simulink model "Simulation_6DOFTesting03"  (R2024a)
settings: Solver=ode4  StartTime=initial_time  StopTime=final_time  FixedStep=timestep  RelTol=1e-3
values from neighbouring files (symbols this model uses):
  aEarth = 0    [CodeTesting_6DOF.m]    (also in Constants_6DOF.m = 6378137; Constants_6DOFTesting.m = 6378137)
  alphaArray = [-30, -25, -20, -15, -10, -5, 0, 5, 10, 15, 20, 25, 30]    [CodeTesting_6DOF.m]    (also in Constants_6DOF.m; Constants_6DOFTesting.m)
  altitudeArray = [0, 1000, 2000, 3000, 4000, 5000, 6000, 7000, 8000, 9000, 10000, 15000, 20000,      25000, 30000, 35000, 40000, 45000, 50000, 55000, 60000]    [CodeTesting_6DOF.m]    (also in Constants_6DOF.m; Constants_6DOFTesting.m)
  bEarth = 0    [CodeTesting_6DOF.m]    (also in Constants_6DOF.m = 6356752.3; Constants_6DOFTesting.m = 6356752.3)
  cD_3DArray = zeros(numAoAs, numMachs, numAltitudes)    [CodeTesting_6DOF.m]    (also in Constants_6DOF.m; Constants_6DOFTesting.m)
  cL_3DArray = zeros(numAoAs, numMachs, numAltitudes)    [CodeTesting_6DOF.m]    (also in Constants_6DOF.m; Constants_6DOFTesting.m)
  densityList = rhoList    [CodeTesting_6DOF.m]    (also in Constants_6DOF.m = usAtmosphere.x_; Constants_6DOFTesting.m = usAtmosphere.x_)
  height0 = 0    [Constants_6DOF.m]    (also in Constants_6DOFTesting.m = 5000)
  heightsList = usAtmosphere.Z    [CodeTesting_6DOF.m]    (also in Constants_6DOF.m; Constants_6DOFTesting.m)
  inertialPitch0 = deg2rad(inertialPitch0)    [Constants_6DOFTesting.m]
  inertialRoll0 = deg2rad(inertialRoll0)    [Constants_6DOFTesting.m]
  inertialYaw0 = deg2rad(inertialYaw0)    [Constants_6DOFTesting.m]
  initQuatVector0 = [e0; e1; e2; e3]    [Constants_6DOFTesting.m]
  Ixx = 10    [CodeTesting_6DOF.m]    (also in Constants_6DOF.m; Constants_6DOFTesting.m = 4.88094462)
  Ixz = 10    [CodeTesting_6DOF.m]    (also in Constants_6DOF.m = 1; Constants_6DOFTesting.m = 4.88094462)
  Iyy = 10    [CodeTesting_6DOF.m]    (also in Constants_6DOF.m; Constants_6DOFTesting.m = 4.88094462)
  Izz = 10    [CodeTesting_6DOF.m]    (also in Constants_6DOF.m; Constants_6DOFTesting.m = 4.88094462)
  latitude0 = pi/4    (= 0.785398163397)    [CodeTesting_6DOF.m]    (also in Constants_6DOF.m = deg2rad(latitude0); Constants_6DOFTesting.m = deg2rad(latitude0))
  longitude0 = pi/4    (= 0.785398163397)    [CodeTesting_6DOF.m]    (also in Constants_6DOF.m = deg2rad(longitude0); Constants_6DOFTesting.m = deg2rad(longitude0))
  m0 = 10    [CodeTesting_6DOF.m]    (also in Constants_6DOF.m = 50; Constants_6DOFTesting.m = 14.5939029)
  machArray = [0.5, 1.0, 1.5, 2.0, 2.5, 3.0, 3.5, 4.0, 4.5, 5.0, 5.5, 6.0, 6.5, 7.0, 7.5, 8.0,      8.5, 9.0, 9.5, 10.0]    [CodeTesting_6DOF.m]    (also in Constants_6DOF.m; Constants_6DOFTesting.m)
  omegaEarth = omega_earth    (= 7.2921159e-05)    [CodeTesting_6DOF.m]    (also in Constants_6DOF.m; Constants_6DOFTesting.m)
  p0Body = deg2rad(p0Body)    [Constants_6DOFTesting.m]
  pitchCharacteristicLength = 0.0    (= 0)    [Constants_6DOFTesting.m]
  q0Body = deg2rad(q0Body)    [Constants_6DOFTesting.m]
  r0Body = deg2rad(r0Body)    [Constants_6DOFTesting.m]
  rEarth = r_earth    (= 6371008.8)    [CodeTesting_6DOF.m]    (also in Constants_6DOF.m; Constants_6DOFTesting.m)
  rollCharacteristicLength = 0.0    (= 0)    [Constants_6DOFTesting.m]
  temperatureList = usAtmosphere.T    [CodeTesting_6DOF.m]    (also in Constants_6DOF.m; Constants_6DOFTesting.m)
  u0Body = 304.8    [Constants_6DOFTesting.m]
  v0Body = 0    [Constants_6DOFTesting.m]
  w0Body = -1 * w0Body    (= 0)    [Constants_6DOFTesting.m]
  wingArea = 0    [CodeTesting_6DOF.m]    (also in Constants_6DOF.m = 50; Constants_6DOFTesting.m = 0.09290304)
  yawCharacteristicLength = 0.0    (= 0)    [Constants_6DOFTesting.m]
undefined symbols (not defined in the file or in its folder): inertialX0, inertialY0, inertialZ0
libraries: simulink_extras x24
(part 1 of 2)
settings Model: Creator=641893  LastModifiedBy=641893

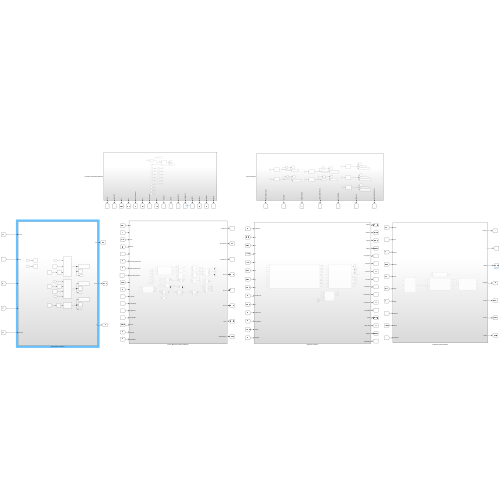
[thumbnail: Simulink's stored preview of the top-level diagram]
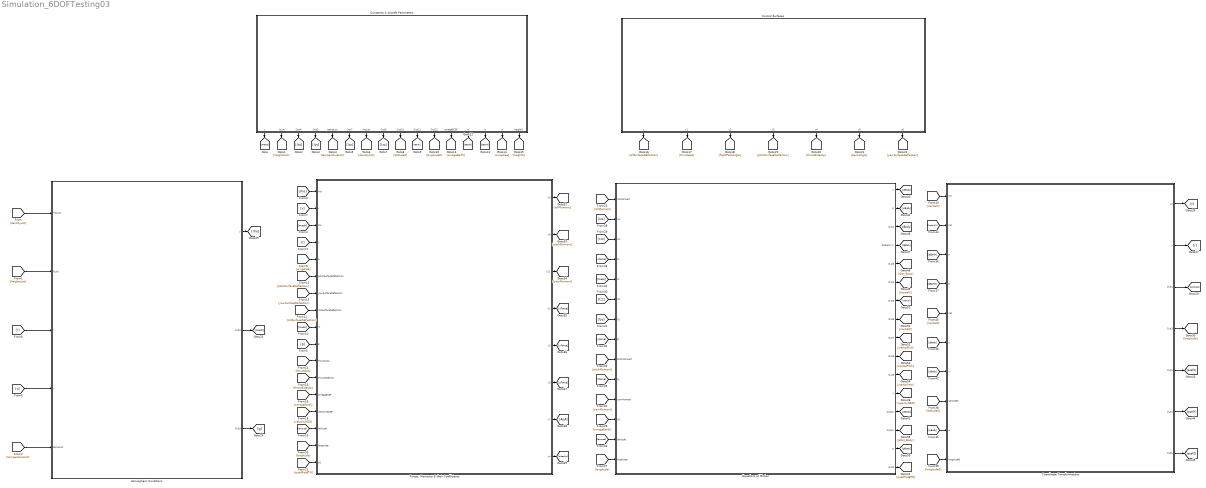
== system Simulation_6DOFTesting03 ==
  Atmospheric Conditions : Subsystem
  Constants & Aircraft Parameters : Subsystem
  Control Surfaces : Subsystem
  Coordinate Transformations : Subsystem
  Equations of Motion : Subsystem
  "Forces, Moments & their Coefficients" : Subsystem
  wires:
  Constants & Aircraft Parameters/1(y) -> [mass]
  Constants & Aircraft Parameters/2(hList) -> [heightsList]
  Constants & Aircraft Parameters/3(Out4) -> [Ixx]
  Constants & Aircraft Parameters/4(Out5) -> [Iyy]
  Constants & Aircraft Parameters/5(tempList) -> [temperatureList]
  Constants & Aircraft Parameters/6(Out7) -> [Izz]
  Constants & Aircraft Parameters/7(rhoList) -> [densityList]
  Constants & Aircraft Parameters/8(Out9) -> [Ixz]
  Constants & Aircraft Parameters/9(Out10) -> [latitude0]
  Constants & Aircraft Parameters/10(Out11) -> [rEarth]
  Constants & Aircraft Parameters/11(Out12) -> [longitude0]
  Constants & Aircraft Parameters/12(omegaECEF) -> [omegaEarth]
  Constants & Aircraft Parameters/13(a) -> [aEarth]
  Constants & Aircraft Parameters/14(b) -> [bEarth]
  Constants & Aircraft Parameters/15(A) -> [wingArea]
  Constants & Aircraft Parameters/16(height0) -> [height0]
  Control Surfaces/1(y) -> [rollSurfaceDeflection]
  Control Surfaces/2(y1) -> [thrustAoA]
  Control Surfaces/4(y3) -> [pitchSurfaceDeflection]
  Control Surfaces/3(y2) -> [flightPathAngle]
  Control Surfaces/5(y4) -> [thrustSideslip]
  Control Surfaces/6(y5) -> [bankAngle]
  Control Surfaces/7(y6) -> [yawSurfaceDeflection]
  [densityList] -> Atmospheric Conditions/1(rhoList)
  [heightsList] -> Atmospheric Conditions/2(hList)
  [temperatureList] -> Atmospheric Conditions/5(tempList)
  Atmospheric Conditions/1(y) -> [rho]
  Atmospheric Conditions/2(Out2) -> [mach]
  Atmospheric Conditions/3(Out3) -> [g]
  [rho] -> "Forces, Moments & their Coefficients"/1(rho)
  [mach] -> "Forces, Moments & their Coefficients"/3(In4)
  [g] -> "Forces, Moments & their Coefficients"/10(g)
  Coordinate Transformations/1(y4) -> [v]
  [v] -> Atmospheric Conditions/4(v)
  [v] -> "Forces, Moments & their Coefficients"/2(v)
  Coordinate Transformations/2(y) -> [r]
  [r] -> Atmospheric Conditions/3(r)
  [wingArea] -> "Forces, Moments & their Coefficients"/5(A)
  [mass] -> "Forces, Moments & their Coefficients"/9(m)
  [rollSurfaceDeflection] -> "Forces, Moments & their Coefficients"/8(rollSurfaceDeflection)
  [pitchSurfaceDeflection] -> "Forces, Moments & their Coefficients"/6(pitchSurfaceDeflection)
  [yawSurfaceDeflection] -> "Forces, Moments & their Coefficients"/7(yawSurfaceDeflection)
  [thrustAoA] -> "Forces, Moments & their Coefficients"/11(thrustAoA)
  [thrustSideslip] -> "Forces, Moments & their Coefficients"/12(thrustSideslip)
  [omegaEarth] -> "Forces, Moments & their Coefficients"/13(omegaECEF)
  [r] -> "Forces, Moments & their Coefficients"/4(y)
  Equations of Motion/12(y) -> [velocityNED]
  [velocityNED] -> "Forces, Moments & their Coefficients"/14(velocityECEF)
  Coordinate Transformations/3(Out1) -> [latitude]
  Coordinate Transformations/4(Out3) -> [longitude]
  [latitude] -> "Forces, Moments & their Coefficients"/15(latitude)
  [longitude] -> "Forces, Moments & their Coefficients"/16(longitude)
  Equations of Motion/16(Out2) -> [quadRotBTN]
  [quadRotBTN] -> "Forces, Moments & their Coefficients"/17(In1)
  "Forces, Moments & their Coefficients"/1(y5) -> [rollMoment]
  "Forces, Moments & their Coefficients"/2(y8) -> [pitchMoment]
  "Forces, Moments & their Coefficients"/3(y11) -> [yawMoment]
  [rollMoment] -> Equations of Motion/1(rollMoment)
  [pitchMoment] -> Equations of Motion/9(pitchMoment)
  [yawMoment] -> Equations of Motion/11(yawMoment)
  [omegaEarth] -> Equations of Motion/12(In1)
  [latitude] -> Equations of Motion/13(latitude)
  [longitude] -> Equations of Motion/14(longitude)
  [Ixx] -> Equations of Motion/2(Ixx)
  [Ixz] -> Equations of Motion/3(Ixz)
  [Izz] -> Equations of Motion/6(Izz)
  [Iyy] -> Equations of Motion/7(Iyy)
  [mass] -> Equations of Motion/5(m)
  "Forces, Moments & their Coefficients"/4(y1) -> [xForce]
  "Forces, Moments & their Coefficients"/5(y2) -> [yForce]
  "Forces, Moments & their Coefficients"/6(y3) -> [zForce]
  [xForce] -> Equations of Motion/4(Fx)
  [yForce] -> Equations of Motion/8(Fy)
  [zForce] -> Equations of Motion/10(Fz)
  "Forces, Moments & their Coefficients"/7(y7) -> [AoA]
  "Forces, Moments & their Coefficients"/8(y4) -> [sideslip]
  [aEarth] -> Coordinate Transformations/3(a)
  [bEarth] -> Coordinate Transformations/4(b)
  [latitude0] -> Coordinate Transformations/8(latitude0)
  [longitude0] -> Coordinate Transformations/10(longitude0)
  Equations of Motion/1(u) -> [uBody]
  Equations of Motion/2(w) -> [wBody]
  [uBody] -> Coordinate Transformations/6(u)
  [wBody] -> Coordinate Transformations/9(w)
  Equations of Motion/13(Out10) -> [vBody]
  [vBody] -> Coordinate Transformations/7(v)
  Equations of Motion/3(Out1) -> [rBody]
  Equations of Motion/4(Radians in) -> [qBody]
  Equations of Motion/5(Out3) -> [rDot_Body]
  Equations of Motion/6(Out4) -> [inertialX]
  Equations of Motion/7(Out5) -> [inertialY]
  Equations of Motion/8(Out6) -> [inertialZ]
  Equations of Motion/9(Out7) -> [inertialRoll]
  Equations of Motion/10(Out8) -> [inertialPitch]
  Equations of Motion/11(Out9) -> [inertialYaw]
  Equations of Motion/14(Out11) -> [pDot_Body]
  Equations of Motion/15(p) -> [pBody]
  [inertialX] -> Coordinate Transformations/1(In1)
  [inertialY] -> Coordinate Transformations/2(In3)
  [inertialZ] -> Coordinate Transformations/5(In8)
  Coordinate Transformations/5(Out2) -> [ecefX]
  Coordinate Transformations/6(Out4) -> [ecefY]
  Coordinate Transformations/7(Out5) -> [ecefZ]

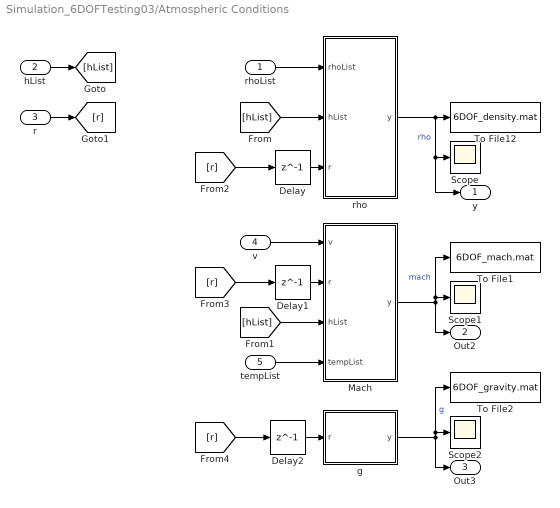
== system Simulation_6DOFTesting03/Atmospheric Conditions ==
  rhoList : Inport
  hList : Inport  Port=2
  r : Inport  Port=3
  v : Inport  Port=4
  tempList : Inport  Port=5
  Delay : Delay  DelayLength=1  InitialCondition=0
  Delay1 : Delay  DelayLength=1  InitialCondition=0
  Delay2 : Delay  DelayLength=1  InitialCondition=0
  Mach : MATLAB Function  TreatAsAtomicUnit=on
  Scope : Scope
  Scope1 : Scope
  Scope2 : Scope
  To File1 : ToFile  Filename=6DOF_mach.mat
  To File12 : ToFile  Filename=6DOF_density.mat
  To File2 : ToFile  Filename=6DOF_gravity.mat
  g : MATLAB Function  TreatAsAtomicUnit=on
  rho : MATLAB Function  TreatAsAtomicUnit=on
  y : Outport
  Out2 : Outport  Port=2
  Out3 : Outport  Port=3
  wires:
  rho/1(y) -> Scope/1, y/1, To File12/1  "rho"
  Mach/1(y) -> To File1/1, Scope1/1, Out2/1  "mach"
  g/1(y) -> Out3/1, To File2/1, Scope2/1  "g"
  v/1 -> Mach/1(v)
  tempList/1 -> Mach/4(tempList)
  r/1 -> [r]
  rhoList/1 -> rho/1(rhoList)
  hList/1 -> [hList]
  [hList] -> rho/2(hList)
  [hList] -> Mach/3(hList)
  Delay/1 -> rho/3(r)
  Delay1/1 -> Mach/2(r)
  Delay2/1 -> g/1(r)
  [r] -> Delay/1
  [r] -> Delay1/1
  [r] -> Delay2/1

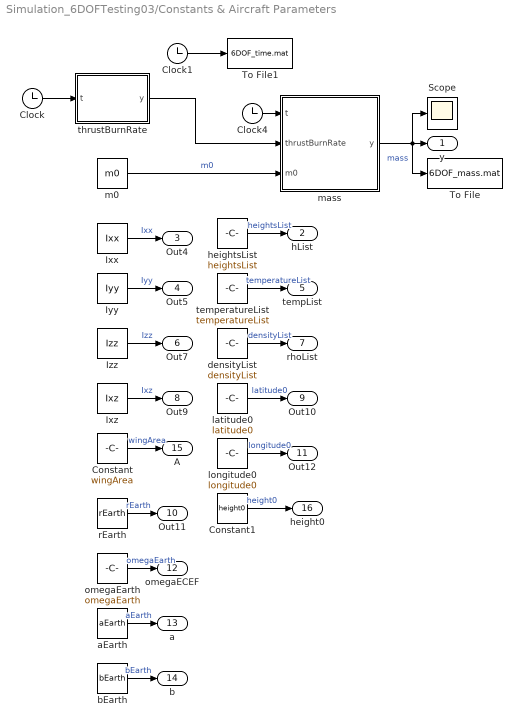
== system Simulation_6DOFTesting03/Constants & Aircraft Parameters ==
  Clock : Clock
  Clock1 : Clock
  Clock4 : Clock
  Constant : Constant  Value=wingArea
  Constant1 : Constant  Value=height0
  Ixx : Constant  Value=Ixx
  Ixz : Constant  Value=Ixz
  Iyy : Constant  Value=Iyy
  Izz : Constant  Value=Izz
  Scope : Scope
  To File : ToFile  Filename=6DOF_mass.mat
  To File1 : ToFile  Filename=6DOF_time.mat
  aEarth : Constant  Value=aEarth
  bEarth : Constant  Value=bEarth
  densityList : Constant  Value=densityList
  heightsList : Constant  Value=heightsList
  latitude0 : Constant  Value=latitude0
  longitude0 : Constant  Value=longitude0
  m0 : Constant  Value=m0
  mass : MATLAB Function  TreatAsAtomicUnit=on
  omegaEarth : Constant  Value=omegaEarth
  rEarth : Constant  Value=rEarth
  temperatureList : Constant  Value=temperatureList
  thrustBurnRate : MATLAB Function  TreatAsAtomicUnit=on
  y : Outport
  hList : Outport  Port=2
  Out4 : Outport  Port=3
  Out5 : Outport  Port=4
  tempList : Outport  Port=5
  Out7 : Outport  Port=6
  rhoList : Outport  Port=7
  Out9 : Outport  Port=8
  Out10 : Outport  Port=9
  Out11 : Outport  Port=10
  Out12 : Outport  Port=11
  omegaECEF : Outport  Port=12
  a : Outport  Port=13
  b : Outport  Port=14
  A : Outport  Port=15
  height0 : Outport  Port=16
  wires:
  m0/1 -> mass/3(m0)  "m0"
  Clock4/1 -> mass/1(t)
  heightsList/1 -> hList/1  "heightsList"
  Clock/1 -> thrustBurnRate/1(t)
  omegaEarth/1 -> omegaECEF/1  "omegaEarth"
  thrustBurnRate/1(y) -> mass/2(thrustBurnRate)
  rEarth/1 -> Out11/1  "rEarth"
  latitude0/1 -> Out10/1  "latitude0"
  mass/1(y) -> To File/1, Scope/1, y/1  "mass"
  aEarth/1 -> a/1  "aEarth"
  densityList/1 -> rhoList/1  "densityList"
  longitude0/1 -> Out12/1  "longitude0"
  bEarth/1 -> b/1  "bEarth"
  Izz/1 -> Out7/1  "Izz"
  Ixz/1 -> Out9/1  "Ixz"
  Ixx/1 -> Out4/1  "Ixx"
  temperatureList/1 -> tempList/1  "temperatureList"
  Iyy/1 -> Out5/1  "Iyy"
  Constant/1 -> A/1  "wingArea"
  Clock1/1 -> To File1/1
  Constant1/1 -> height0/1  "height0"

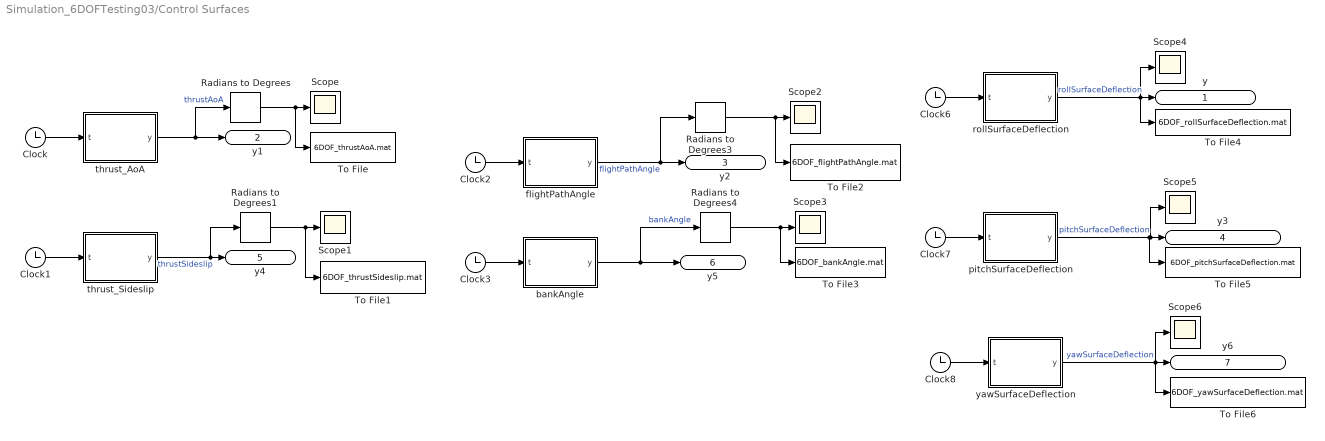
== system Simulation_6DOFTesting03/Control Surfaces ==
  Clock{,1..3,6..8} (7 alike) : Clock
  Radians to Degrees{,1,3..4} (4 alike) : simulink_extras/Transformations/Radians to Degrees
  Scope{,1..6} (7 alike) : Scope
  To File : ToFile  Filename=6DOF_thrustAoA.mat
  To File1 : ToFile  Filename=6DOF_thrustSideslip.mat
  To File2 : ToFile  Filename=6DOF_flightPathAngle.mat
  To File3 : ToFile  Filename=6DOF_bankAngle.mat
  To File4 : ToFile  Filename=6DOF_rollSurfaceDeflection.mat
  To File5 : ToFile  Filename=6DOF_pitchSurfaceDeflection.mat
  To File6 : ToFile  Filename=6DOF_yawSurfaceDeflection.mat
  bankAngle : MATLAB Function  TreatAsAtomicUnit=on
  flightPathAngle : MATLAB Function  TreatAsAtomicUnit=on
  pitchSurfaceDeflection : MATLAB Function  TreatAsAtomicUnit=on
  rollSurfaceDeflection : MATLAB Function  TreatAsAtomicUnit=on
  thrust_AoA : MATLAB Function  TreatAsAtomicUnit=on
  thrust_Sideslip : MATLAB Function  TreatAsAtomicUnit=on
  yawSurfaceDeflection : MATLAB Function  TreatAsAtomicUnit=on
  y : Outport
  y1 : Outport  Port=2
  y2 : Outport  Port=3
  y3 : Outport  Port=4
  y4 : Outport  Port=5
  y5 : Outport  Port=6
  y6 : Outport  Port=7
  wires:
  Clock8/1 -> yawSurfaceDeflection/1(t)
  rollSurfaceDeflection/1(y) -> Scope4/1, y/1, To File4/1  "rollSurfaceDeflection"
  Clock1/1 -> thrust_Sideslip/1(t)
  bankAngle/1(y) -> Radians to Degrees4/1, y5/1  "bankAngle"
  Clock6/1 -> rollSurfaceDeflection/1(t)
  Clock7/1 -> pitchSurfaceDeflection/1(t)
  pitchSurfaceDeflection/1(y) -> To File5/1, Scope5/1, y3/1  "pitchSurfaceDeflection"
  Clock2/1 -> flightPathAngle/1(t)
  thrust_AoA/1(y) -> Radians to Degrees/1, y1/1  "thrustAoA"
  Clock/1 -> thrust_AoA/1(t)
  Clock3/1 -> bankAngle/1(t)
  thrust_Sideslip/1(y) -> Radians to Degrees1/1, y4/1  "thrustSideslip"
  flightPathAngle/1(y) -> Radians to Degrees3/1, y2/1  "flightPathAngle"
  yawSurfaceDeflection/1(y) -> Scope6/1, y6/1, To File6/1  "yawSurfaceDeflection"
  Radians to Degrees/1 -> To File/1, Scope/1
  Radians to Degrees1/1 -> To File1/1, Scope1/1
  Radians to Degrees3/1 -> To File2/1, Scope2/1
  Radians to Degrees4/1 -> Scope3/1, To File3/1

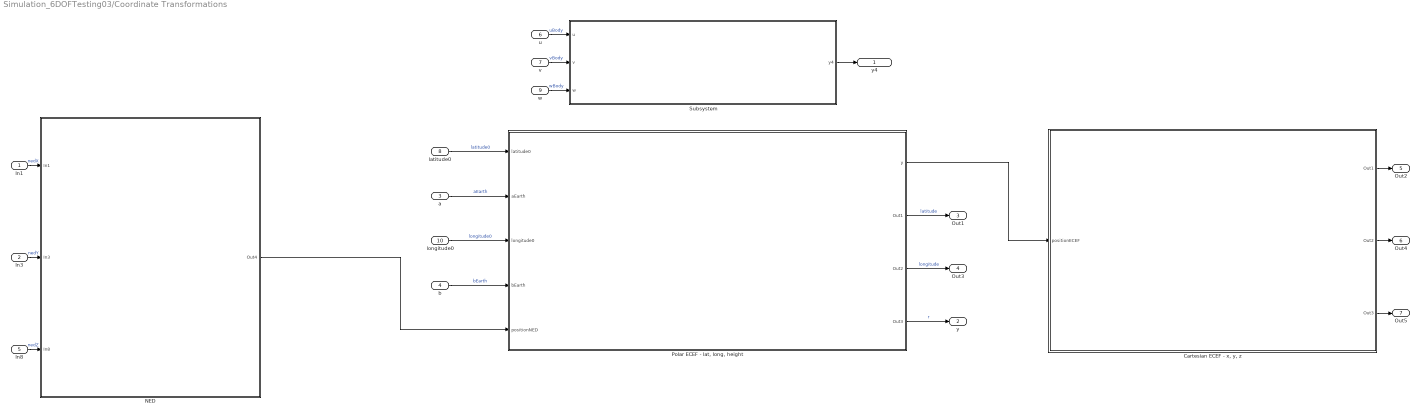
== system Simulation_6DOFTesting03/Coordinate Transformations ==
  In1 : Inport
  In3 : Inport  Port=2
  a : Inport  Port=3
  b : Inport  Port=4
  In8 : Inport  Port=5
  u : Inport  Port=6
  v : Inport  Port=7
  latitude0 : Inport  Port=8
  w : Inport  Port=9
  longitude0 : Inport  Port=10
  "Cartesian ECEF - x, y, z" : Subsystem
  NED : Subsystem
  "Polar ECEF - lat, long, height" : Subsystem
  Subsystem : Subsystem
  y4 : Outport
  y : Outport  Port=2
  Out1 : Outport  Port=3
  Out3 : Outport  Port=4
  Out2 : Outport  Port=5
  Out4 : Outport  Port=6
  Out5 : Outport  Port=7
  wires:
  b/1 -> "Polar ECEF - lat, long, height"/4(bEarth)  "bEarth"
  longitude0/1 -> "Polar ECEF - lat, long, height"/3(longitude0)  "longitude0"
  latitude0/1 -> "Polar ECEF - lat, long, height"/1(latitude0)  "latitude0"
  a/1 -> "Polar ECEF - lat, long, height"/2(aEarth)  "aEarth"
  NED/1(Out4) -> "Polar ECEF - lat, long, height"/5(positionNED)
  In1/1 -> NED/1(In1)  "nedX"
  In3/1 -> NED/2(In3)  "nedY"
  In8/1 -> NED/3(In8)  "nedZ"
  "Polar ECEF - lat, long, height"/1(y) -> "Cartesian ECEF - x, y, z"/1(positionECEF)
  u/1 -> Subsystem/1(u)  "uBody"
  v/1 -> Subsystem/2(v)  "vBody"
  w/1 -> Subsystem/3(w)  "wBody"
  Subsystem/1(y4) -> y4/1
  "Polar ECEF - lat, long, height"/3(Out2) -> Out3/1  "longitude"
  "Polar ECEF - lat, long, height"/2(Out1) -> Out1/1  "latitude"
  "Cartesian ECEF - x, y, z"/3(Out3) -> Out5/1
  "Cartesian ECEF - x, y, z"/2(Out2) -> Out4/1
  "Cartesian ECEF - x, y, z"/1(Out1) -> Out2/1
  "Polar ECEF - lat, long, height"/4(Out3) -> y/1  "r"

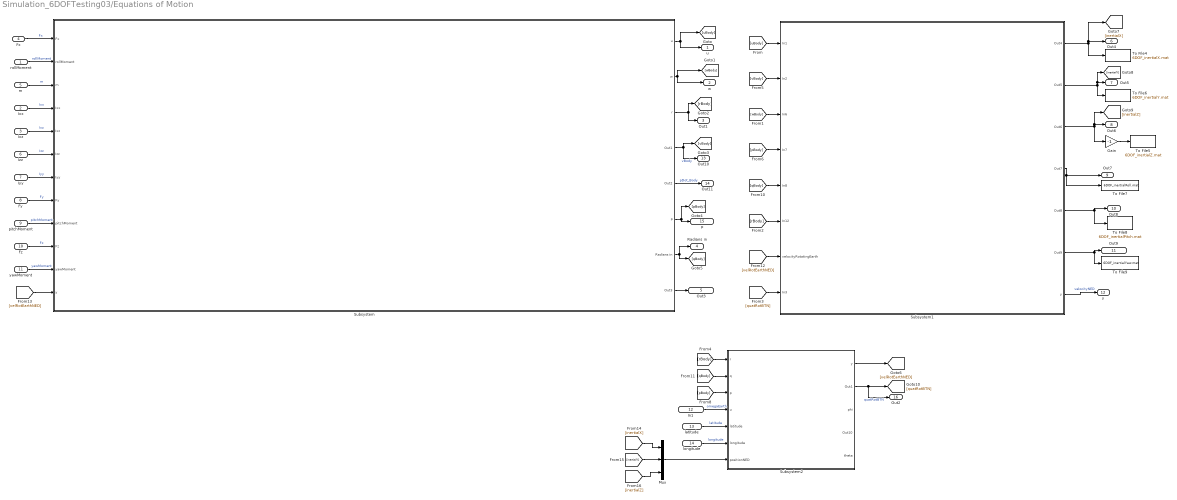
== system Simulation_6DOFTesting03/Equations of Motion ==
  rollMoment : Inport
  Ixx : Inport  Port=2
  Ixz : Inport  Port=3
  Fx : Inport  Port=4
  m : Inport  Port=5
  Izz : Inport  Port=6
  Iyy : Inport  Port=7
  Fy : Inport  Port=8
  pitchMoment : Inport  Port=9
  Fz : Inport  Port=10
  yawMoment : Inport  Port=11
  In1 : Inport  Port=12
  latitude : Inport  Port=13
  longitude : Inport  Port=14
  Gain : Gain  Gain=-1
  Mux : Mux  Inputs=3
  Subsystem : Subsystem
  Subsystem1 : Subsystem
  Subsystem2 : Subsystem
  To File4 : ToFile  Filename=6DOF_inertialX.mat
  To File5 : ToFile  Filename=6DOF_inertialZ.mat
  To File6 : ToFile  Filename=6DOF_inertialY.mat
  To File7 : ToFile  Filename=6DOF_inertialRoll.mat
  To File8 : ToFile  Filename=6DOF_inertialPitch.mat
  To File9 : ToFile  Filename=6DOF_inertialYaw.mat
  u : Outport
  w : Outport  Port=2
  Out1 : Outport  Port=3
  Radians in : Outport  Port=4
  Out3 : Outport  Port=5
  Out4 : Outport  Port=6
  Out5 : Outport  Port=7
  Out6 : Outport  Port=8
  Out7 : Outport  Port=9
  Out8 : Outport  Port=10
  Out9 : Outport  Port=11
  y : Outport  Port=12
  Out10 : Outport  Port=13
  Out11 : Outport  Port=14
  p : Outport  Port=15
  Out2 : Outport  Port=16
  wires:
  Fx/1 -> Subsystem/1(Fx)  "Fx"
  rollMoment/1 -> Subsystem/2(rollMoment)  "rollMoment"
  m/1 -> Subsystem/3(m)  "m"
  Ixx/1 -> Subsystem/4(Ixx)  "Ixx"
  Ixz/1 -> Subsystem/5(Ixz)  "Ixz"
  Izz/1 -> Subsystem/6(Izz)  "Izz"
  Iyy/1 -> Subsystem/7(Iyy)  "Iyy"
  Fy/1 -> Subsystem/8(Fy)  "Fy"
  pitchMoment/1 -> Subsystem/9(pitchMoment)  "pitchMoment"
  Fz/1 -> Subsystem/10(Fz)  "Fz"
  yawMoment/1 -> Subsystem/11(yawMoment)  "yawMoment"
  Subsystem/1(u) -> [uBody], u/1
  Subsystem/2(w) -> [wBody], w/1
  Subsystem/3(r) -> [rBody], Out1/1
  Subsystem/8(Out3) -> Out3/1
  Subsystem1/1(Out4) -> Out4/1, [inertialX], To File4/1
  Subsystem1/2(Out5) -> Out5/1, [inertialY], To File6/1
  Subsystem1/3(Out6) -> Out6/1, [inertialZ], Gain/1
  Subsystem1/4(Out7) -> To File7/1, Out7/1
  Subsystem1/6(Out9) -> Out9/1, To File9/1
  In1/1 -> Subsystem2/4(u)  "omegaEarth"
  Subsystem2/1(y) -> [velRotEarthNED]
  latitude/1 -> Subsystem2/5(latitude)  "latitude"
  longitude/1 -> Subsystem2/6(longitude)  "longitude"
  Mux/1 -> Subsystem2/7(positionNED)
  Gain/1 -> To File5/1
  Subsystem1/7(y) -> y/1  "velocityNED"
  [uBody] -> Subsystem1/1(In1)
  [wBody] -> Subsystem1/3(In6)
  [rBody] -> Subsystem1/6(In12)
  [rBody] -> Subsystem2/1(r)
  Subsystem/4(Out1) -> [vBody], Out10/1  "vBody"
  [vBody] -> Subsystem1/2(In2)
  Subsystem/6(p) -> p/1, [pBody]
  [pBody] -> Subsystem1/4(In7)
  [pBody] -> Subsystem2/3(p)
  Subsystem/5(Out2) -> Out11/1  "pDot_Body"
  Subsystem/7(Radians in) -> [qBody], Radians in/1
  [qBody] -> Subsystem1/5(In8)
  [qBody] -> Subsystem2/2(q)
  [velRotEarthNED] -> Subsystem1/7(velocityRotatingEarth)
  [velRotEarthNED] -> Subsystem/12(y)
  [inertialX] -> Mux/1
  [inertialY] -> Mux/2
  [inertialZ] -> Mux/3
  Subsystem1/5(Out8) -> Out8/1, To File8/1
  Subsystem2/2(Out1) -> Out2/1, [quatRotBTN]  "quatRotBTN"
  [quatRotBTN] -> Subsystem1/8(In3)

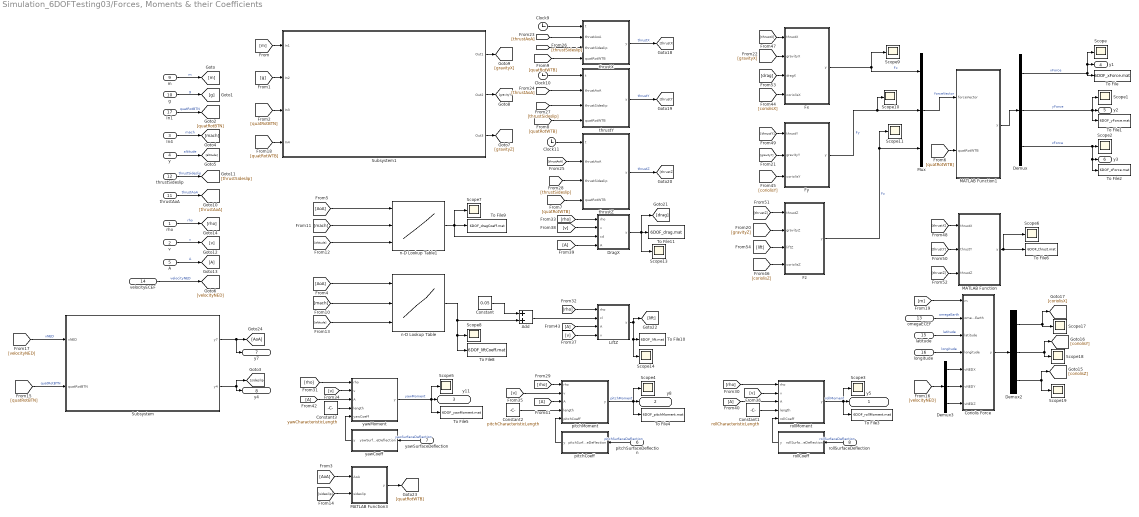
== system Simulation_6DOFTesting03/Forces, Moments & their Coefficients ==
  rho : Inport
  v : Inport  Port=2
  In4 : Inport  Port=3
  y : Inport  Port=4
  A : Inport  Port=5
  pitchSurfaceDeflection : Inport  Port=6
  yawSurfaceDeflection : Inport  Port=7
  rollSurfaceDeflection : Inport  Port=8
  m : Inport  Port=9
  g : Inport  Port=10
  thrustAoA : Inport  Port=11
  thrustSideslip : Inport  Port=12
  omegaECEF : Inport  Port=13
  velocityECEF : Inport  Port=14
  latitude : Inport  Port=15
  longitude : Inport  Port=16
  In1 : Inport  Port=17
  Add : Sum
  Clock10 : Clock
  Clock11 : Clock
  Clock9 : Clock
  Constant : Constant  Value=0.05
  Constant1 : Constant  Value=rollCharacteristicLength
  Constant2 : Constant  Value=pitchCharacteristicLength
  Constant3 : Constant  Value=yawCharacteristicLength
  Coriolis Force : MATLAB Function  TreatAsAtomicUnit=on
  Demux : Demux  Outputs=3
  Demux2 : Demux  Outputs=3
  Demux3 : Demux  Outputs=3
  DragX : MATLAB Function  TreatAsAtomicUnit=on
  From{39..43} (5 alike) : From
  Fx : MATLAB Function  TreatAsAtomicUnit=on
  Fy : MATLAB Function  TreatAsAtomicUnit=on
  Fz : MATLAB Function  TreatAsAtomicUnit=on
  Goto13 : Goto
  LiftZ : MATLAB Function  TreatAsAtomicUnit=on
  MATLAB Function : MATLAB Function  TreatAsAtomicUnit=on
  MATLAB Function1 : MATLAB Function  TreatAsAtomicUnit=on
  MATLAB Function3 : MATLAB Function  TreatAsAtomicUnit=on
  Mux : Mux  Inputs=3
  Scope{,1..11,13..14,17..19} (17 alike) : Scope
  Subsystem : Subsystem
  Subsystem1 : Subsystem
  To File : ToFile  Filename=6DOF_xForce.mat
  To File1 : ToFile  Filename=6DOF_yForce.mat
  To File10 : ToFile  Filename=6DOF_lift.mat
  To File11 : ToFile  Filename=6DOF_drag.mat
  To File2 : ToFile  Filename=6DOF_zForce.mat
  To File3 : ToFile  Filename=6DOF_rollMoment.mat
  To File4 : ToFile  Filename=6DOF_pitchMoment.mat
  To File5 : ToFile  Filename=6DOF_yawMoment.mat
  To File6 : ToFile  Filename=6DOF_thrust.mat
  To File8 : ToFile  Filename=6DOF_liftCoeff.mat
  To File9 : ToFile  Filename=6DOF_dragCoeff.mat
  n-D Lookup Table : Lookup_n-D  NumberOfTableDimensions=3  BreakpointsForDimension1=alphaArray  BreakpointsForDimension2=machArray  BreakpointsForDimension3=altitudeArray  IndexSearchMethod=Linear search  Table=cL_3DArray  InterpMethod=Linear Lagrange  InternalRulePriority=Speed  RndMeth=Simplest
      settings: InputPortMap=u0,u1,u2
  n-D Lookup Table1 : Lookup_n-D  NumberOfTableDimensions=3  BreakpointsForDimension1=alphaArray  BreakpointsForDimension2=machArray  BreakpointsForDimension3=altitudeArray  IndexSearchMethod=Linear search  Table=cD_3DArray  InterpMethod=Linear Lagrange  InternalRulePriority=Speed  RndMeth=Simplest
      settings: InputPortMap=u0,u1,u2
  pitchCoeff : MATLAB Function  TreatAsAtomicUnit=on
  pitchMoment : MATLAB Function  TreatAsAtomicUnit=on
  rollCoeff : MATLAB Function  TreatAsAtomicUnit=on
  rollMoment : MATLAB Function  TreatAsAtomicUnit=on
  thrustX : MATLAB Function  TreatAsAtomicUnit=on
  thrustY : MATLAB Function  TreatAsAtomicUnit=on
  thrustZ : MATLAB Function  TreatAsAtomicUnit=on
  yawCoeff : MATLAB Function  TreatAsAtomicUnit=on
  yawMoment : MATLAB Function  TreatAsAtomicUnit=on
  y5 : Outport
  y8 : Outport  Port=2
  y11 : Outport  Port=3
  y1 : Outport  Port=4
  y2 : Outport  Port=5
  y3 : Outport  Port=6
  y7 : Outport  Port=7
  y4 : Outport  Port=8
  wires:
  Clock11/1 -> thrustZ/1(t)
  n-D Lookup Table/1 -> Add/2, To File8/1, Scope8/1
  LiftZ/1(y) -> [lift], Scope14/1, To File10/1
  n-D Lookup Table1/1 -> DragX/3(cd), Scope7/1, To File9/1
  v/1 -> [v]  "v"
  DragX/1(y) -> Scope13/1, To File11/1, [drag]
  rollMoment/1(y) -> Scope3/1, y5/1, To File3/1  "rollMoment"
  yawSurfaceDeflection/1 -> yawCoeff/1(yawSurfaceDeflection)  "yawSurfaceDeflection"
  yawMoment/1(y) -> To File5/1, Scope5/1, y11/1  "yawMoment"
  Clock9/1 -> thrustX/1(t)
  rho/1 -> [rho]  "rho"
  Clock10/1 -> thrustY/1(t)
  rollSurfaceDeflection/1 -> rollCoeff/1(rollSurfaceDeflection)  "rollSurfaceDeflection"
  A/1 -> Goto13/1  "A"
  thrustAoA/1 -> [thrustAoA]  "thrustAoA"
  In4/1 -> [mach]  "mach"
  thrustSideslip/1 -> [thrustSideslip]  "thrustSideslip"
  pitchMoment/1(y) -> Scope4/1, y8/1, To File4/1  "pitchMoment"
  pitchSurfaceDeflection/1 -> pitchCoeff/1(pitchSurfaceDeflection)  "pitchSurfaceDeflection"
  pitchCoeff/1(y) -> pitchMoment/5(pitchCoeff)
  rollCoeff/1(y) -> rollMoment/5(rollCoeff)
  yawCoeff/1(y) -> yawMoment/5(yawCoeff)
  Fx/1(y) -> Mux/1, Scope9/1  "Fx"
  thrustX/1(y) -> [thrustX]  "thrustX"
  Fy/1(y) -> Scope10/1, Mux/2  "Fy"
  Fz/1(y) -> Scope11/1, Mux/3  "Fz"
  MATLAB Function/1(y) -> Scope6/1, To File6/1
  Add/1 -> LiftZ/2(cl)
  Constant/1 -> Add/1
  Demux/1 -> Scope/1, y1/1, To File/1  "xForce"
  Demux/2 -> To File1/1, y2/1, Scope1/1  "yForce"
  Demux/3 -> To File2/1, y3/1, Scope2/1  "zForce"
  Mux/1 -> MATLAB Function1/1(forceVector)  "forceVector"
  MATLAB Function1/1(y) -> Demux/1
  g/1 -> [g]  "g"
  m/1 -> [m]  "m"
  Demux2/1 -> [coriolisX], Scope17/1
  Demux2/2 -> [coriolisY], Scope18/1
  Demux2/3 -> [coriolisZ], Scope19/1
  longitude/1 -> Coriolis Force/4(longitude)  "longitude"
  latitude/1 -> Coriolis Force/3(latitude)  "latitude"
  omegaECEF/1 -> Coriolis Force/2(omegaEarth)  "omegaEarth"
  Coriolis Force/1(y) -> Demux2/1
  Demux3/1 -> Coriolis Force/5(vNEDX)
  Demux3/2 -> Coriolis Force/6(vNEDY)
  Demux3/3 -> Coriolis Force/7(vNEDZ)
  velocityECEF/1 -> [velocityNED]  "velocityNED"
  Constant1/1 -> rollMoment/4(length)
  Constant2/1 -> pitchMoment/4(length)
  Constant3/1 -> yawMoment/4(length)
  In1/1 -> [quatRotBTN]  "quatRotBTN"
  [AoA] -> n-D Lookup Table/1
  [AoA] -> n-D Lookup Table1/1
  [mach] -> n-D Lookup Table/2
  [mach] -> n-D Lookup Table1/2
  y/1 -> [altitude]  "altitude"
  [altitude] -> n-D Lookup Table1/3
  [altitude] -> n-D Lookup Table/3
  [m] -> Coriolis Force/1(m)
  [gravityZ] -> Fz/2(gravityZ)
  [gravityY] -> Fy/2(gravityY)
  [gravityX] -> Fx/2(gravityX)
  [thrustAoA] -> thrustX/2(thrustAoA)
  [thrustAoA] -> thrustY/2(thrustAoA)
  [thrustAoA] -> thrustZ/2(thrustAoA)
  [thrustSideslip] -> thrustX/3(thrustSideslip)
  [thrustSideslip] -> thrustY/3(thrustSideslip)
  [thrustSideslip] -> thrustZ/3(thrustSideslip)
  [rho] -> DragX/1(rho)
  [rho] -> LiftZ/1(rho)
  [rho] -> rollMoment/1(rho)
  [rho] -> pitchMoment/1(rho)
  [rho] -> yawMoment/1(rho)
  [v] -> LiftZ/4(v)
  [v] -> rollMoment/2(v)
  [v] -> pitchMoment/2(v)
  [v] -> yawMoment/2(v)
  From43/1 -> LiftZ/3(A)
  From39/1 -> DragX/4(A)
  From40/1 -> rollMoment/3(A)
  From41/1 -> pitchMoment/3(A)
  From42/1 -> yawMoment/3(A)
  [v] -> DragX/2(v)
  [coriolisX] -> Fx/4(coriolisX)
  [coriolisY] -> Fy/3(coriolisY)
  [coriolisZ] -> Fz/4(coriolisZ)
  [thrustX] -> Fx/1(thrustX)
  [thrustX] -> MATLAB Function/1(thrustX)
  thrustY/1(y) -> [thrustY]  "thrustY"
  [thrustY] -> Fy/1(thrustY)
  [thrustY] -> MATLAB Function/2(thrustY)
  thrustZ/1(y) -> [thrustZ]  "thrustZ"
  [thrustZ] -> Fz/1(thrustZ)
  [thrustZ] -> MATLAB Function/3(thrustZ)
  [drag] -> Fx/3(dragX)
  [lift] -> Fz/3(liftZ)
  [sideslip] -> MATLAB Function3/2(sideslip)
  [AoA] -> MATLAB Function3/1(AoA)
  MATLAB Function3/1(y) -> [quatRotWTB]
  [quatRotWTB] -> thrustZ/4(quatRotWTB)
  [quatRotWTB] -> thrustY/4(quatRotWTB)
  [quatRotWTB] -> thrustX/4(quatRotWTB)
  [quatRotWTB] -> MATLAB Function1/2(quatRotWTB)
  Subsystem/1(y7) -> y7/1, [AoA]
  Subsystem/2(y4) -> y4/1, [sideslip]
  [velocityNED] -> Subsystem/1(vNED)  "vNED"
  [quatRotBTN] -> Subsystem/2(quatRotBTN)  "quatRotBTN"
  [velocityNED] -> Demux3/1
  Subsystem1/1(Out1) -> [gravityX]
  Subsystem1/2(Out2) -> [gravityY]
  Subsystem1/3(Out3) -> [gravityZ]
  [m] -> Subsystem1/1(In1)
  [g] -> Subsystem1/2(In2)
  [quatRotBTN] -> Subsystem1/3(In3)
  [quatRotWTB] -> Subsystem1/4(In4)

== system Simulation_6DOFTesting03/Coordinate Transformations/Cartesian ECEF - x, y, z ==
  positionECEF : Inport
  Demux2 : Demux  Outputs=3
  MATLAB Function : MATLAB Function  TreatAsAtomicUnit=on
  MATLAB Function4 : MATLAB Function  TreatAsAtomicUnit=on
  Scope{,2,7..8,10} (5 alike) : Scope
  To File10 : ToFile  Filename=6DOF_ecefX.mat
  To File7 : ToFile  Filename=6DOF_ecefY.mat
  To File8 : ToFile  Filename=6DOF_ecefZ.mat
  Out1 : Outport
  Out2 : Outport  Port=2
  Out3 : Outport  Port=3
  wires:
  positionECEF/1 -> MATLAB Function4/1(positionECEF), MATLAB Function/1(u), Demux2/1
  Demux2/2 -> Scope7/1, To File7/1, Out2/1  "ecefY"
  Demux2/3 -> Out3/1, To File8/1, Scope8/1  "ecefZ"
  MATLAB Function4/1(y) -> Scope2/1  "r"
  Demux2/1 -> Out1/1, Scope10/1, To File10/1  "ecefX"
  MATLAB Function/1(y) -> Scope/1

== system Simulation_6DOFTesting03/Coordinate Transformations/NED ==
  In1 : Inport
  In3 : Inport  Port=2
  In8 : Inport  Port=3
  Gain : Gain  Gain=-1
  Mux : Mux  Inputs=3
  Scope4 : Scope
  Scope5 : Scope
  Scope6 : Scope
  To File4 : ToFile  Filename=6DOF_nedX.mat
  To File5 : ToFile  Filename=6DOF_nedY.mat
  To File6 : ToFile  Filename=6DOF_nedZ.mat
  Out4 : Outport
  wires:
  In8/1 -> Gain/1
  In1/1 -> [nedX], Scope4/1, To File4/1
  Mux/1 -> Out4/1  "positionNED"
  Gain/1 -> Scope6/1, To File6/1, [nedZ]  "nedZ"
  In3/1 -> [nedY], Scope5/1, To File5/1
  [nedX] -> Mux/1
  [nedY] -> Mux/2
  [nedZ] -> Mux/3

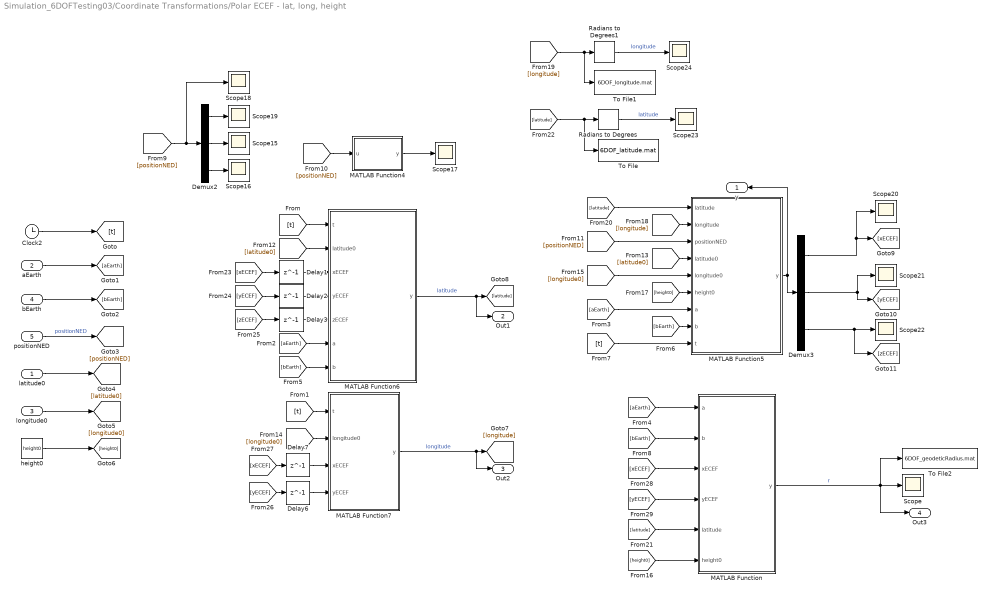
== system Simulation_6DOFTesting03/Coordinate Transformations/Polar ECEF - lat, long, height ==
  latitude0 : Inport
  aEarth : Inport  Port=2
  longitude0 : Inport  Port=3
  bEarth : Inport  Port=4
  positionNED : Inport  Port=5
  Clock2 : Clock
  Delay{1..3,6..7} (5 alike) : Delay  DelayLength=1  InitialCondition=0
  Demux2 : Demux  Outputs=3
  Demux3 : Demux  Outputs=3
  MATLAB Function : MATLAB Function  TreatAsAtomicUnit=on
  MATLAB Function4 : MATLAB Function  TreatAsAtomicUnit=on
  MATLAB Function5 : MATLAB Function  TreatAsAtomicUnit=on
  MATLAB Function6 : MATLAB Function  TreatAsAtomicUnit=on
  MATLAB Function7 : MATLAB Function  TreatAsAtomicUnit=on
  Radians to Degrees : simulink_extras/Transformations/Radians to Degrees
  Radians to Degrees1 : simulink_extras/Transformations/Radians to Degrees
  Scope{,15..24} (11 alike) : Scope
  To File : ToFile  Filename=6DOF_latitude.mat
  To File1 : ToFile  Filename=6DOF_longitude.mat
  To File2 : ToFile  Filename=6DOF_geodeticRadius.mat
  height0 : Constant  Value=height0
  y : Outport
  Out1 : Outport  Port=2
  Out2 : Outport  Port=3
  Out3 : Outport  Port=4
  wires:
  latitude0/1 -> [latitude0]
  bEarth/1 -> [bEarth]
  aEarth/1 -> [aEarth]
  longitude0/1 -> [longitude0]
  height0/1 -> [height0]
  MATLAB Function4/1(y) -> Scope17/1
  Demux2/1 -> Scope19/1
  Demux2/2 -> Scope15/1
  Demux2/3 -> Scope16/1
  MATLAB Function5/1(y) -> y/1, Demux3/1
  Demux3/1 -> Scope20/1, [xECEF]
  Demux3/2 -> [yECEF], Scope21/1
  Clock2/1 -> [t]
  Demux3/3 -> [zECEF], Scope22/1
  MATLAB Function6/1(y) -> Out1/1, [latitude]  "latitude"
  MATLAB Function7/1(y) -> Out2/1, [longitude]  "longitude"
  Radians to Degrees/1 -> Scope23/1  "latitude"
  Radians to Degrees1/1 -> Scope24/1  "longitude"
  MATLAB Function/1(y) -> To File2/1, Scope/1, Out3/1  "r"
  [t] -> MATLAB Function6/1(t)
  [t] -> MATLAB Function7/1(t)
  [aEarth] -> MATLAB Function6/6(a)
  [aEarth] -> MATLAB Function5/7(a)
  [aEarth] -> MATLAB Function/1(a)
  [bEarth] -> MATLAB Function6/7(b)
  [bEarth] -> MATLAB Function5/8(b)
  [t] -> MATLAB Function5/9(t)
  [bEarth] -> MATLAB Function/2(b)
  positionNED/1 -> [positionNED]  "positionNED"
  [positionNED] -> Demux2/1, Scope18/1
  [positionNED] -> MATLAB Function4/1(u)
  [positionNED] -> MATLAB Function5/3(positionNED)
  [latitude0] -> MATLAB Function6/2(latitude0)
  [latitude0] -> MATLAB Function5/4(latitude0)
  [longitude0] -> MATLAB Function7/2(longitude0)
  [longitude0] -> MATLAB Function5/5(longitude0)
  [height0] -> MATLAB Function/6(height0)
  [height0] -> MATLAB Function5/6(height0)
  [longitude] -> MATLAB Function5/2(longitude)
  [longitude] -> To File1/1, Radians to Degrees1/1
  [latitude] -> MATLAB Function5/1(latitude)
  [latitude] -> MATLAB Function/5(latitude)
  [latitude] -> To File/1, Radians to Degrees/1
  Delay1/1 -> MATLAB Function6/3(xECEF)
  [xECEF] -> Delay1/1
  Delay2/1 -> MATLAB Function6/4(yECEF)
  [yECEF] -> Delay2/1
  Delay3/1 -> MATLAB Function6/5(zECEF)
  [zECEF] -> Delay3/1
  Delay6/1 -> MATLAB Function7/4(yECEF)
  [yECEF] -> Delay6/1
  Delay7/1 -> MATLAB Function7/3(xECEF)
  [xECEF] -> Delay7/1
  [xECEF] -> MATLAB Function/3(xECEF)
  [yECEF] -> MATLAB Function/4(yECEF)

== system Simulation_6DOFTesting03/Coordinate Transformations/Subsystem ==
  u : Inport
  v : Inport  Port=2
  w : Inport  Port=3
  Scope1 : Scope
  To File1 : ToFile  Filename=6DOF_velocity.mat
  velocity : MATLAB Function  TreatAsAtomicUnit=on
  y4 : Outport
  wires:
  v/1 -> velocity/2(v)
  velocity/1(y) -> Scope1/1, To File1/1, y4/1  "velocity"
  u/1 -> velocity/1(u)
  w/1 -> velocity/3(w)

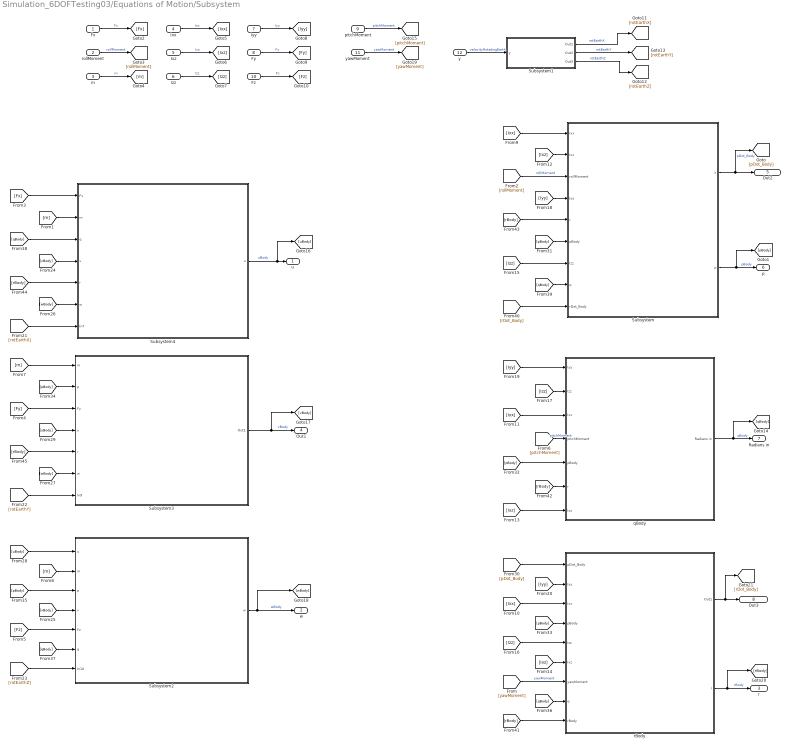
== system Simulation_6DOFTesting03/Equations of Motion/Subsystem ==
  Fx : Inport
  rollMoment : Inport  Port=2
  m : Inport  Port=3
  Ixx : Inport  Port=4
  Ixz : Inport  Port=5
  Izz : Inport  Port=6
  Iyy : Inport  Port=7
  Fy : Inport  Port=8
  pitchMoment : Inport  Port=9
  Fz : Inport  Port=10
  yawMoment : Inport  Port=11
  y : Inport  Port=12
  Subsystem : Subsystem
  Subsystem1 : Subsystem
  Subsystem2 : Subsystem
  Subsystem3 : Subsystem
  Subsystem4 : Subsystem
  qBody : Subsystem
  rBody : Subsystem
  u : Outport
  w : Outport  Port=2
  r : Outport  Port=3
  Out1 : Outport  Port=4
  Out2 : Outport  Port=5
  p : Outport  Port=6
  Radians in : Outport  Port=7
  Out3 : Outport  Port=8
  wires:
  Ixx/1 -> [Ixx]  "Ixx"
  Ixz/1 -> [Ixz]  "Ixz"
  Iyy/1 -> [Iyy]  "Iyy"
  Izz/1 -> [Izz]  "Izz"
  m/1 -> [m]  "m"
  yawMoment/1 -> [yawMoment]  "yawMoment"
  rBody/2(r) -> [rBody], r/1  "rBody"
  qBody/1(Radians in) -> Radians in/1, [qBody]  "qBody"
  pitchMoment/1 -> [pitchMoment]  "pitchMoment"
  rollMoment/1 -> [rollMoment]  "rollMoment"
  rBody/1(Out1) -> [rDot_Body], Out3/1
  y/1 -> Subsystem1/1(y)  "velocityRotatingEarth"
  Fz/1 -> [Fz]  "Fz"
  Subsystem1/3(Out3) -> [rotEarthZ]  "rotEarthZ"
  Fy/1 -> [Fy]  "Fy"
  Subsystem1/2(Out2) -> [rotEarthY]  "rotEarthY"
  Fx/1 -> [Fx]  "Fx"
  Subsystem1/1(Out1) -> [rotEarthX]  "rotEarthX"
  Subsystem4/1(u) -> [uBody], u/1  "uBody"
  [yawMoment] -> rBody/7(yawMoment)  "yawMoment"
  [pitchMoment] -> qBody/4(pitchMoment)  "pitchMoment"
  [rollMoment] -> Subsystem/3(rollMoment)  "rollMoment"
  [Fx] -> Subsystem4/1(Fx)
  [Fy] -> Subsystem3/3(Fy)
  [Fz] -> Subsystem2/5(Fz)
  [m] -> Subsystem4/2(m)
  [m] -> Subsystem3/1(m)
  [m] -> Subsystem2/2(m)
  [Ixx] -> Subsystem/1(Ixx)
  [Ixx] -> qBody/3(Ixx)
  [Ixx] -> rBody/3(Ixx)
  [Ixz] -> Subsystem/2(Ixz)
  [Ixz] -> qBody/7(Ixz)
  [Ixz] -> rBody/6(Ixz)
  [Izz] -> Subsystem/7(Izz)
  [Izz] -> qBody/2(Izz)
  [Izz] -> rBody/5(Izz)
  [Iyy] -> rBody/2(Iyy)
  [Iyy] -> qBody/1(Iyy)
  [Iyy] -> Subsystem/4(Iyy)
  [rotEarthX] -> Subsystem4/7(In7)
  [rotEarthY] -> Subsystem3/7(In9)
  [rotEarthZ] -> Subsystem2/7(In10)
  Subsystem3/1(Out1) -> Out1/1, [vBody]  "vBody"
  [vBody] -> Subsystem4/4(v)
  [vBody] -> Subsystem2/4(v)
  Subsystem2/1(w) -> [wBody], w/1  "wBody"
  [wBody] -> Subsystem3/6(w)
  [wBody] -> Subsystem4/6(w)
  [uBody] -> Subsystem3/4(u)
  [uBody] -> Subsystem2/1(u)
  Subsystem/1(y) -> Out2/1, [pDot_Body]  "pDot_Body"
  [pDot_Body] -> rBody/1(pDot_Body)
  [pBody] -> Subsystem2/3(p)
  [pBody] -> Subsystem3/2(p)
  Subsystem/2(p) -> p/1, [pBody]  "pBody"
  [pBody] -> Subsystem/6(pBody)
  [pBody] -> qBody/5(pBody)
  [pBody] -> rBody/4(pBody)
  [qBody] -> Subsystem/8(q)
  [qBody] -> rBody/8(q)
  [qBody] -> Subsystem4/3(q)
  [qBody] -> Subsystem2/6(q)
  [rDot_Body] -> Subsystem/9(rDot_Body)
  [rBody] -> rBody/9(rBody)
  [rBody] -> qBody/6(r)
  [rBody] -> Subsystem/5(r)
  [rBody] -> Subsystem4/5(r)
  [rBody] -> Subsystem3/5(r)

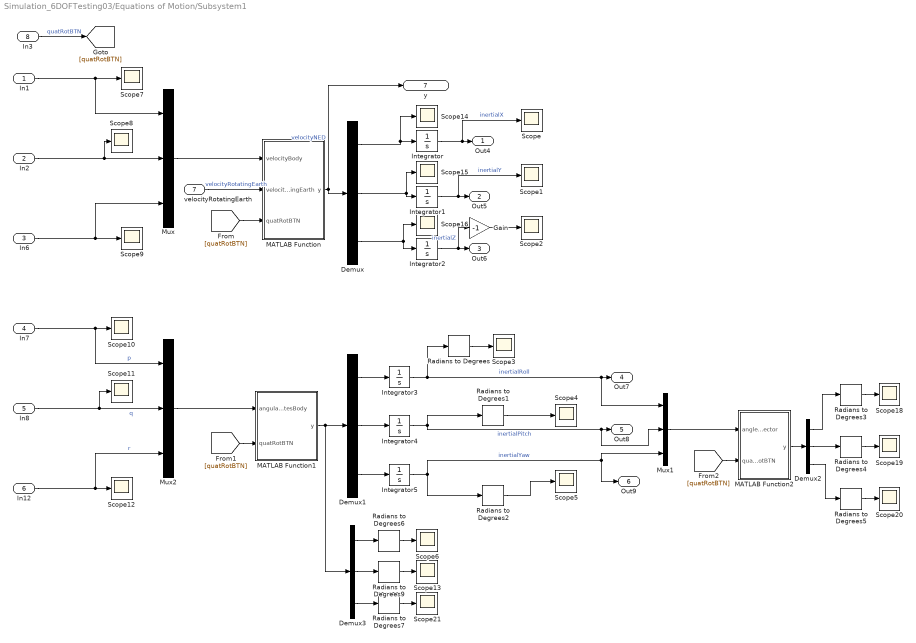
== system Simulation_6DOFTesting03/Equations of Motion/Subsystem1 ==
  In1 : Inport
  In2 : Inport  Port=2
  In6 : Inport  Port=3
  In7 : Inport  Port=4
  In8 : Inport  Port=5
  In12 : Inport  Port=6
  velocityRotatingEarth : Inport  Port=7
  In3 : Inport  Port=8
  Demux{,1..3} (4 alike) : Demux  Outputs=3
  Gain : Gain  Gain=-1
  Integrator : Integrator  InitialCondition=inertialX0
  Integrator1 : Integrator  InitialCondition=inertialY0
  Integrator2 : Integrator  InitialCondition=inertialZ0
  Integrator3 : Integrator  InitialCondition=inertialRoll0
  Integrator4 : Integrator  InitialCondition=inertialPitch0
  Integrator5 : Integrator  InitialCondition=inertialYaw0
  MATLAB Function : MATLAB Function  TreatAsAtomicUnit=on
  MATLAB Function1 : MATLAB Function  TreatAsAtomicUnit=on
  MATLAB Function2 : MATLAB Function  TreatAsAtomicUnit=on
  Mux : Mux  Inputs=3
  Mux1 : Mux  Inputs=3
  Mux2 : Mux  Inputs=3
  Radians to Degrees{,1..7,9} (9 alike) : simulink_extras/Transformations/Radians to Degrees
  Scope{,1..16,18..21} (21 alike) : Scope
  Out4 : Outport
  Out5 : Outport  Port=2
  Out6 : Outport  Port=3
  Out7 : Outport  Port=4
  Out8 : Outport  Port=5
  Out9 : Outport  Port=6
  y : Outport  Port=7
  wires:
  In6/1 -> Scope9/1, Mux/3
  Demux1/1 -> Integrator3/1
  Demux1/3 -> Integrator5/1
  Integrator4/1 -> Radians to Degrees1/1, Mux1/2, Out8/1  "inertialPitch"
  Mux/1 -> MATLAB Function/1(velocityBody)
  Integrator/1 -> Scope/1, Out4/1  "inertialX"
  Integrator5/1 -> Radians to Degrees2/1, Mux1/3, Out9/1  "inertialYaw"
  Demux/1 -> Scope14/1, Integrator/1
  Demux1/2 -> Integrator4/1
  MATLAB Function/1(y) -> Demux/1, y/1  "velocityNED"
  Demux/2 -> Integrator1/1, Scope15/1
  Integrator3/1 -> Radians to Degrees/1, Mux1/1, Out7/1  "inertialRoll"
  Demux/3 -> Scope16/1, Integrator2/1
  Mux2/1 -> MATLAB Function1/1(angularRatesBody)
  In12/1 -> Mux2/3, Scope12/1  "r"
  MATLAB Function1/1(y) -> Demux1/1, Demux3/1
  Integrator2/1 -> Gain/1, Out6/1  "inertialZ"
  Integrator1/1 -> Scope1/1, Out5/1  "inertialY"
  In8/1 -> Scope11/1, Mux2/2  "q"
  In7/1 -> Scope10/1, Mux2/1  "p"
  In2/1 -> Scope8/1, Mux/2
  In1/1 -> Scope7/1, Mux/1
  velocityRotatingEarth/1 -> MATLAB Function/2(velocityRotatingEarth)  "velocityRotatingEarth"
  Gain/1 -> Scope2/1
  Radians to Degrees/1 -> Scope3/1
  Radians to Degrees1/1 -> Scope4/1
  Radians to Degrees2/1 -> Scope5/1
  Mux1/1 -> MATLAB Function2/1(angleVector)
  MATLAB Function2/1(y) -> Demux2/1
  Demux2/2 -> Radians to Degrees4/1
  Demux2/3 -> Radians to Degrees5/1
  Radians to Degrees3/1 -> Scope18/1
  Demux2/1 -> Radians to Degrees3/1
  Radians to Degrees4/1 -> Scope19/1
  Radians to Degrees5/1 -> Scope20/1
  Radians to Degrees9/1 -> Scope13/1
  Demux3/2 -> Radians to Degrees9/1
  Radians to Degrees6/1 -> Scope6/1
  Demux3/1 -> Radians to Degrees6/1
  Radians to Degrees7/1 -> Scope21/1
  Demux3/3 -> Radians to Degrees7/1
  In3/1 -> [quatRotBTN]  "quatRotBTN"
  [quatRotBTN] -> MATLAB Function1/2(quatRotBTN)
  [quatRotBTN] -> MATLAB Function/3(quatRotBTN)
  [quatRotBTN] -> MATLAB Function2/2(quatRotBTN)

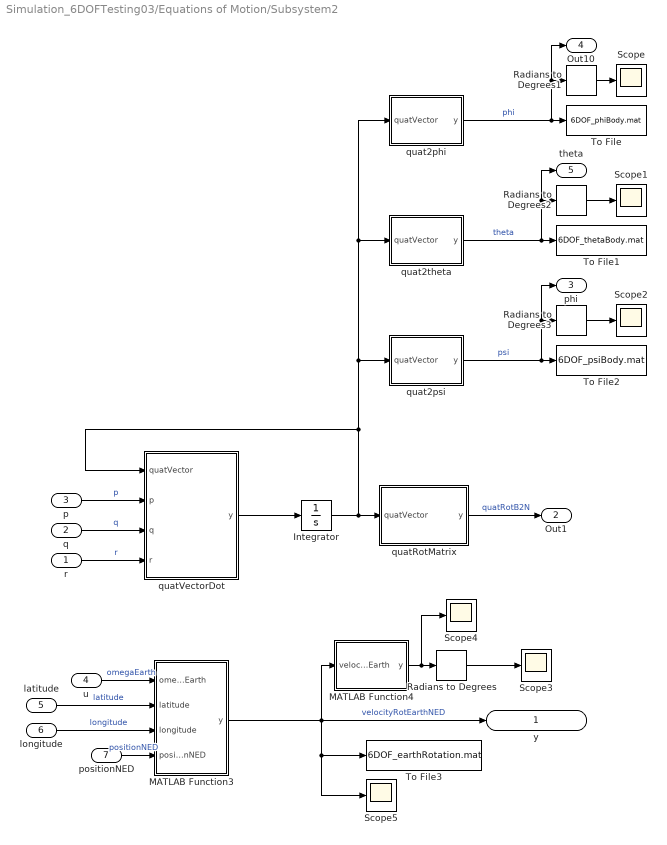
== system Simulation_6DOFTesting03/Equations of Motion/Subsystem2 ==
  r : Inport
  q : Inport  Port=2
  p : Inport  Port=3
  u : Inport  Port=4
  latitude : Inport  Port=5
  longitude : Inport  Port=6
  positionNED : Inport  Port=7
  Integrator : Integrator  InitialCondition=initQuatVector0
  MATLAB Function3 : MATLAB Function  TreatAsAtomicUnit=on
  MATLAB Function4 : MATLAB Function  TreatAsAtomicUnit=on
  Radians to Degrees{,1..3} (4 alike) : simulink_extras/Transformations/Radians to Degrees
  Scope{,1..5} (6 alike) : Scope
  To File : ToFile  Filename=6DOF_phiBody.mat
  To File1 : ToFile  Filename=6DOF_thetaBody.mat
  To File2 : ToFile  Filename=6DOF_psiBody.mat
  To File3 : ToFile  Filename=6DOF_earthRotation.mat
  quat2phi : MATLAB Function  TreatAsAtomicUnit=on
  quat2psi : MATLAB Function  TreatAsAtomicUnit=on
  quat2theta : MATLAB Function  TreatAsAtomicUnit=on
  quatRotMatrix : MATLAB Function  TreatAsAtomicUnit=on
  quatVectorDot : MATLAB Function  TreatAsAtomicUnit=on
  y : Outport
  Out1 : Outport  Port=2
  phi : Outport  Port=3
  Out10 : Outport  Port=4
  theta : Outport  Port=5
  wires:
  u/1 -> MATLAB Function3/1(omegaEarth)  "omegaEarth"
  MATLAB Function3/1(y) -> Scope5/1, To File3/1, y/1, MATLAB Function4/1(velocityRotatingEarth)  "velocityRotEarthNED"
  latitude/1 -> MATLAB Function3/2(latitude)  "latitude"
  longitude/1 -> MATLAB Function3/3(longitude)  "longitude"
  MATLAB Function4/1(y) -> Radians to Degrees/1, Scope4/1
  Radians to Degrees/1 -> Scope3/1
  positionNED/1 -> MATLAB Function3/4(positionNED)  "positionNED"
  p/1 -> quatVectorDot/2(p)  "p"
  q/1 -> quatVectorDot/3(q)  "q"
  r/1 -> quatVectorDot/4(r)  "r"
  quatVectorDot/1(y) -> Integrator/1
  Integrator/1 -> quat2theta/1(quatVector), quat2phi/1(quatVector), quat2psi/1(quatVector), quatVectorDot/1(quatVector), quatRotMatrix/1(quatVector)
  quatRotMatrix/1(y) -> Out1/1  "quatRotB2N"
  quat2phi/1(y) -> Out10/1, Radians to Degrees1/1, To File/1  "phi"
  Radians to Degrees1/1 -> Scope/1
  quat2theta/1(y) -> theta/1, Radians to Degrees2/1, To File1/1  "theta"
  Radians to Degrees2/1 -> Scope1/1
  quat2psi/1(y) -> phi/1, Radians to Degrees3/1, To File2/1  "psi"
  Radians to Degrees3/1 -> Scope2/1

== system Simulation_6DOFTesting03/Forces, Moments & their Coefficients/Subsystem ==
  vNED : Inport
  quatRotBTN : Inport  Port=2
  AoA1 : MATLAB Function  TreatAsAtomicUnit=on
  Demux : Demux  Outputs=3
  Demux1 : Demux  Outputs=3
  MATLAB Function : MATLAB Function  TreatAsAtomicUnit=on
  Radians to Degrees2 : simulink_extras/Transformations/Radians to Degrees
  Radians to Degrees5 : simulink_extras/Transformations/Radians to Degrees
  Scope20 : Scope
  Scope21 : Scope
  To File12 : ToFile  Filename=6DOF_sideslip.mat
  To File7 : ToFile  Filename=6DOF_AoA.mat
  sideslipAngle1 : MATLAB Function  TreatAsAtomicUnit=on
  y7 : Outport
  y4 : Outport  Port=2
  wires:
  sideslipAngle1/1(y) -> y4/1, Radians to Degrees2/1  "sideslipAngle"
  Radians to Degrees5/1 -> Scope20/1, To File7/1
  AoA1/1(y) -> y7/1, Radians to Degrees5/1  "AoA"
  Radians to Degrees2/1 -> To File12/1, Scope21/1
  vNED/1 -> MATLAB Function/1(vNED)  "vNED"
  quatRotBTN/1 -> MATLAB Function/2(quatRotBTN)  "quatRotBTN"
  Demux/2 -> sideslipAngle1/2(v)
  Demux/1 -> sideslipAngle1/1(u)
  Demux/3 -> sideslipAngle1/3(w)
  MATLAB Function/1(y) -> Demux1/1, Demux/1
  Demux1/2 -> AoA1/2(v)
  Demux1/1 -> AoA1/1(u)
  Demux1/3 -> AoA1/3(w)

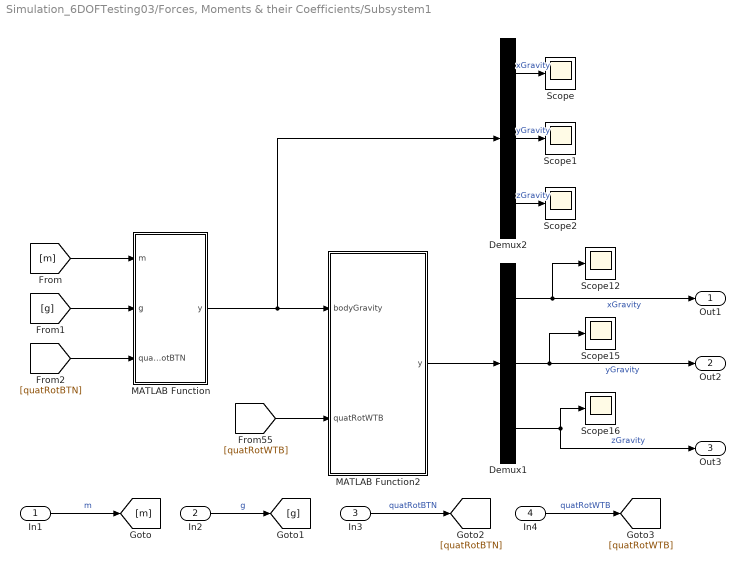
== system Simulation_6DOFTesting03/Forces, Moments & their Coefficients/Subsystem1 ==
  In1 : Inport
  In2 : Inport  Port=2
  In3 : Inport  Port=3
  In4 : Inport  Port=4
  Demux1 : Demux  Outputs=3
  Demux2 : Demux  Outputs=3
  MATLAB Function : MATLAB Function  TreatAsAtomicUnit=on
  MATLAB Function2 : MATLAB Function  TreatAsAtomicUnit=on
  Scope{,1..2,12,15..16} (6 alike) : Scope
  Out1 : Outport
  Out2 : Outport  Port=2
  Out3 : Outport  Port=3
  wires:
  [quatRotWTB] -> MATLAB Function2/2(quatRotWTB)
  Demux1/2 -> Out2/1, Scope15/1  "yGravity"
  Demux1/3 -> Out3/1, Scope16/1  "zGravity"
  Demux1/1 -> Out1/1, Scope12/1  "xGravity"
  MATLAB Function2/1(y) -> Demux1/1
  In1/1 -> [m]  "m"
  In2/1 -> [g]  "g"
  In3/1 -> [quatRotBTN]  "quatRotBTN"
  In4/1 -> [quatRotWTB]  "quatRotWTB"
  MATLAB Function/1(y) -> MATLAB Function2/1(bodyGravity), Demux2/1
  [m] -> MATLAB Function/1(m)
  [g] -> MATLAB Function/2(g)
  [quatRotBTN] -> MATLAB Function/3(quatRotBTN)
  Demux2/1 -> Scope/1  "xGravity"
  Demux2/2 -> Scope1/1  "yGravity"
  Demux2/3 -> Scope2/1  "zGravity"

== system Simulation_6DOFTesting03/Equations of Motion/Subsystem/Subsystem ==
  Ixx : Inport
  Ixz : Inport  Port=2
  rollMoment : Inport  Port=3
  Iyy : Inport  Port=4
  r : Inport  Port=5
  pBody : Inport  Port=6
  Izz : Inport  Port=7
  q : Inport  Port=8
  rDot_Body : Inport  Port=9
  Delay2 : Delay  DelayLength=1  InitialCondition=0
  Integrator3 : Integrator  InitialCondition=p0Body
  Radians to Degrees : simulink_extras/Transformations/Radians to Degrees
  Scope12 : Scope
  Scope6 : Scope
  To File6 : ToFile  Filename=6DOF_pBody.mat
  pDot_Body : MATLAB Function  TreatAsAtomicUnit=on
  y : Outport
  p : Outport  Port=2
  wires:
  Delay2/1 -> y/1, Scope12/1, Integrator3/1  "pDot_Body"
  rDot_Body/1 -> pDot_Body/4(rDot_Body)
  pBody/1 -> pDot_Body/9(p)
  Iyy/1 -> pDot_Body/6(Iyy)
  Radians to Degrees/1 -> Scope6/1, To File6/1
  pDot_Body/1(y) -> Delay2/1
  Ixz/1 -> pDot_Body/3(Ixz)
  Izz/1 -> pDot_Body/5(Izz)
  r/1 -> pDot_Body/8(r)
  Integrator3/1 -> p/1, Radians to Degrees/1  "pBody"
  rollMoment/1 -> pDot_Body/1(rollMoment)
  Ixx/1 -> pDot_Body/2(Ixx)
  q/1 -> pDot_Body/7(q)

== system Simulation_6DOFTesting03/Equations of Motion/Subsystem/Subsystem1 ==
  y : Inport
  Demux : Demux  Outputs=3
  Out1 : Outport
  Out2 : Outport  Port=2
  Out3 : Outport  Port=3
  wires:
  y/1 -> Demux/1
  Demux/1 -> Out1/1  "rotEarthX"
  Demux/3 -> Out3/1  "rotEarthZ"
  Demux/2 -> Out2/1  "rotEarthY"

== system Simulation_6DOFTesting03/Equations of Motion/Subsystem/Subsystem2 ==
  u : Inport
  m : Inport  Port=2
  p : Inport  Port=3
  v : Inport  Port=4
  Fz : Inport  Port=5
  q : Inport  Port=6
  In10 : Inport  Port=7
  Delay5 : Delay  DelayLength=1  InitialCondition=0
  Integrator2 : Integrator  InitialCondition=w0Body
  Scope2 : Scope
  Sum2 : Sum  Inputs=|++
  To File2 : ToFile  Filename=6DOF_wBody.mat
  wDot_Body : MATLAB Function  TreatAsAtomicUnit=on
  w : Outport
  wires:
  p/1 -> wDot_Body/5(p)
  Fz/1 -> wDot_Body/1(Fz)
  In10/1 -> Sum2/2  "rotEarthZ"
  m/1 -> wDot_Body/2(m)
  wDot_Body/1(y) -> Integrator2/1
  Sum2/1 -> Delay5/1  "wBody"
  Integrator2/1 -> Sum2/1  "wWind"
  Delay5/1 -> To File2/1, Scope2/1, w/1  "wBody"
  u/1 -> wDot_Body/4(u)
  v/1 -> wDot_Body/6(v)
  q/1 -> wDot_Body/3(q)

== system Simulation_6DOFTesting03/Equations of Motion/Subsystem/Subsystem3 ==
  m : Inport
  p : Inport  Port=2
  Fy : Inport  Port=3
  u : Inport  Port=4
  r : Inport  Port=5
  w : Inport  Port=6
  In9 : Inport  Port=7
  Delay4 : Delay  DelayLength=1  InitialCondition=0
  Integrator1 : Integrator  InitialCondition=v0Body
  Sum1 : Sum  Inputs=|++
  To File1 : ToFile  Filename=6DOF_vBody.mat
  vDot_Body : MATLAB Function  TreatAsAtomicUnit=on
  Out1 : Outport
  wires:
  Delay4/1 -> To File1/1, Out1/1  "vBody"
  Sum1/1 -> Delay4/1  "vBody"
  u/1 -> vDot_Body/6(u)
  Integrator1/1 -> Sum1/1  "vWind"
  vDot_Body/1(y) -> Integrator1/1
  Fy/1 -> vDot_Body/1(Fy)
  m/1 -> vDot_Body/2(m)
  p/1 -> vDot_Body/3(p)
  w/1 -> vDot_Body/4(w)
  r/1 -> vDot_Body/5(r)
  In9/1 -> Sum1/2  "rotEarthY"

== system Simulation_6DOFTesting03/Equations of Motion/Subsystem/Subsystem4 ==
  Fx : Inport
  m : Inport  Port=2
  q : Inport  Port=3
  v : Inport  Port=4
  r : Inport  Port=5
  w : Inport  Port=6
  In7 : Inport  Port=7
  Delay1 : Delay  DelayLength=1  InitialCondition=0
  Integrator : Integrator  InitialCondition=u0Body
  Scope : Scope
  Sum : Sum  Inputs=|++
  To File : ToFile  Filename=6DOF_uBody.mat
  uDot_Body : MATLAB Function  TreatAsAtomicUnit=on
  u : Outport
  wires:
  Sum/1 -> Delay1/1  "uBody"
  v/1 -> uDot_Body/4(v)
  m/1 -> uDot_Body/2(m)
  uDot_Body/1(y) -> Integrator/1
  Delay1/1 -> Scope/1, To File/1, u/1  "uBody"
  Integrator/1 -> Sum/1  "uWind"
  Fx/1 -> uDot_Body/1(Fx)
  q/1 -> uDot_Body/5(q)
  In7/1 -> Sum/2  "rotEarthX"
  w/1 -> uDot_Body/6(w)
  r/1 -> uDot_Body/3(r)

== system Simulation_6DOFTesting03/Equations of Motion/Subsystem/qBody ==
  Iyy : Inport
  Izz : Inport  Port=2
  Ixx : Inport  Port=3
  pitchMoment : Inport  Port=4
  pBody : Inport  Port=5
  r : Inport  Port=6
  Ixz : Inport  Port=7
  Delay : Delay  DelayLength=1  InitialCondition=0
  Integrator4 : Integrator  InitialCondition=q0Body
  Radians to Degrees1 : simulink_extras/Transformations/Radians to Degrees
  Scope13 : Scope
  Scope7 : Scope
  To File7 : ToFile  Filename=6DOF_qBody.mat
  qDot_Body : MATLAB Function  TreatAsAtomicUnit=on
  Radians in : Outport
  wires:
  qDot_Body/1(y) -> Integrator4/1, Scope13/1
  Ixz/1 -> qDot_Body/7(Ixz)
  Delay/1 -> Radians to Degrees1/1, Radians in/1  "q_Body"
  Ixx/1 -> qDot_Body/4(Ixx)
  Radians to Degrees1/1 -> To File7/1, Scope7/1
  Iyy/1 -> qDot_Body/2(Iyy)
  Integrator4/1 -> Delay/1  "qBody"
  pBody/1 -> qDot_Body/5(p)
  Izz/1 -> qDot_Body/3(Izz)
  pitchMoment/1 -> qDot_Body/1(pitchMoment)
  r/1 -> qDot_Body/6(r)

== system Simulation_6DOFTesting03/Equations of Motion/Subsystem/rBody ==
  pDot_Body : Inport
  Iyy : Inport  Port=2
  Ixx : Inport  Port=3
  pBody : Inport  Port=4
  Izz : Inport  Port=5
  Ixz : Inport  Port=6
  yawMoment : Inport  Port=7
  q : Inport  Port=8
  rBody : Inport  Port=9
  Delay3 : Delay  DelayLength=1  InitialCondition=0
  Integrator5 : Integrator  InitialCondition=r0Body
  Radians to Degrees2 : simulink_extras/Transformations/Radians to Degrees
  Scope10 : Scope
  To File10 : ToFile  Filename=6DOF_rBody.mat
  rDot_Body : MATLAB Function  TreatAsAtomicUnit=on
  Out1 : Outport
  r : Outport  Port=2
  wires:
  Delay3/1 -> Out1/1, Integrator5/1  "rDot_Body"
  Radians to Degrees2/1 -> Scope10/1, To File10/1
  Integrator5/1 -> Radians to Degrees2/1, r/1  "rBody"
  rDot_Body/1(y) -> Delay3/1
  Ixz/1 -> rDot_Body/3(Ixz)
  Iyy/1 -> rDot_Body/6(Iyy)
  yawMoment/1 -> rDot_Body/1(yawMoment)
  pBody/1 -> rDot_Body/7(p)
  Izz/1 -> rDot_Body/2(Izz)
  pDot_Body/1 -> rDot_Body/4(pDot_Body)
  q/1 -> rDot_Body/8(q)
  rBody/1 -> rDot_Body/9(r)
  Ixx/1 -> rDot_Body/5(Ixx)

== matlab function Simulation_6DOFTesting03/Forces, Moments & their Coefficients/thrustY ==
  data: t input; y output; thrustAoA input; thrustSideslip input; quatRotWTB input
function y = fcn(t, thrustAoA, thrustSideslip,quatRotWTB)

thrust = 0;

thrust = thrust * cos(thrustAoA) * sin(thrustSideslip);

thrustVector = [0; thrust; 0];

thrustWind = inv(quatRotWTB) * thrustVector;

thrustWindY = thrustWind(2);

y = thrustWindY;
